simulink model "Vorlage_Prozessgut_Gruppen3"  (R2023b)
settings: Solver=ode3  StartTime=0.0  StopTime=200  FixedStep=0.01  RelTol=1e-3  EnableMultiTasking=on
undefined symbols (not defined in the file): MaxFlaschen
libraries: simulink x10
settings Model: Creator=merz  LastModifiedBy=JCP
settings SolverCC: ZeroCrossAlgorithm=Non-adaptive  AlgebraicLoopSolver=TrustRegion  AutoInsertRateTranBlk=on
settings DataIOCC: LimitDataPoints=on  SaveFormat=Array  SignalLoggingSaveFormat=ModelDataLogs  ReturnWorkspaceOutputs=off  SignalLoggingName=sigsOut
settings OptimizationCC: ExpressionDepthLimit=2147483647  InitFltsAndDblsToZero=on  LifeSpan=inf
settings DebuggingCC: SaveWithParameterizedLinksMsg=none  UnderspecifiedInitializationDetection=Classic  MergeDetectMultiDrivingBlocksExec=none  SignalResolutionControl=TryResolveAllWithWarning  MultiTaskDSMMsg=warning  MultiTaskCondExecSysMsg=none  FcnCallInpInsideContextMsg=warning  UnconnectedInputMsg=warning  UnconnectedOutputMsg=warning  UnconnectedLineMsg=warning  StateNameClashWarn=warning  SFUnexpectedBacktrackingDiag=warning  SFNoUnconditionalDefaultTransitionDiag=warning  SFExecutionAtInitializationDiag=none  ArithmeticOperatorsInVariantConditions=warning
settings HardwareCC: ProdBitPerPointer=32  ProdBitPerSizeT=32  ProdBitPerPtrDiffT=32  ProdLargestAtomicFloat=None  ProdIntDivRoundTo=Undefined  ProdEndianess=Unspecified  ProdWordSize=32  ProdHWDeviceType=32-bit Generic  TargetUnknown=on
settings ModelReferenceCC: EnableRefExpFcnMdlSchedulingChecks=on  PropagateSignalLabelsOutOfModel=off
settings RTWCC: DLArmComputeVersion=19.05
settings CodeAppCC: StateflowObjectComments=on
settings GRTTargetCC: TargetFcnLib=ansi_tfl_tmw.mat  TargetLangStandard=C89/C90 (ANSI)  ModelReferenceCompliant=off  CombineOutputUpdateFcns=off  MatFileLogging=off  GRTInterface=on
settings ConfigComp: CovMetricSettings=dw  CovSaveCumulativeToWorkspaceVar=on  CovSaveSingleToWorkspaceVar=on

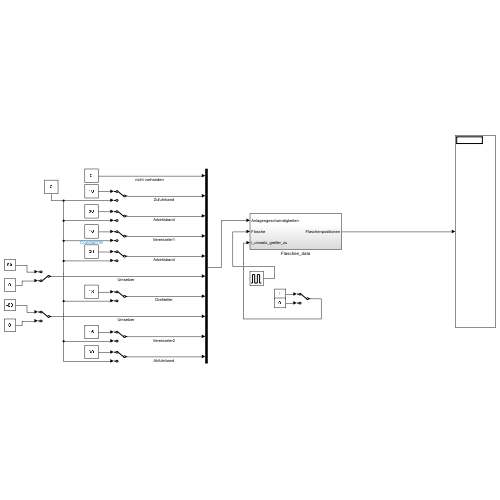
[thumbnail: Simulink's stored preview of the top-level diagram]
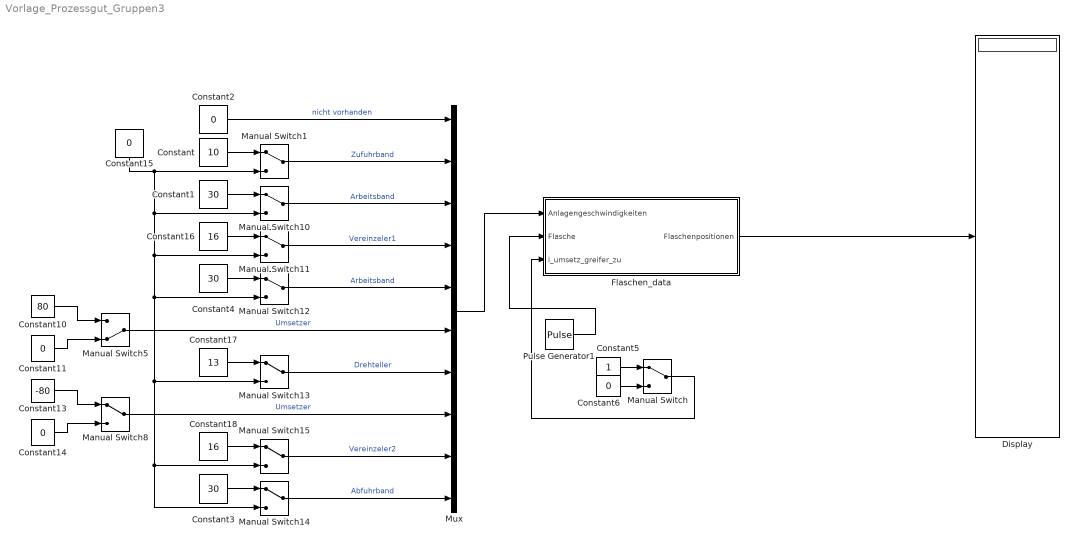
== system Vorlage_Prozessgut_Gruppen3 ==
  Constant : Constant  Value=10
  Constant1 : Constant  Value=30
  Constant10 : Constant  Value=80
  Constant{2,6,11,14..15} (5 alike) : Constant  Value=0
  Constant13 : Constant  Value=-80
  Constant16 : Constant  Value=16
  Constant17 : Constant  Value=13
  Constant18 : Constant  Value=16
  Constant3 : Constant  Value=30
  Constant4 : Constant  Value=30
  Constant5 : Constant
  Display : Display
  Flaschen_data : Subsystem
  Manual Switch{,1,8,10..15} (9 alike) : ManualSwitch
  Manual Switch5 : ManualSwitch  CurrentSetting=0
  Mux : Mux  Inputs=10
  Pulse Generator1 : DiscretePulseGenerator  PulseType=Time based  Period=15  PulseWidth=5
  wires:
  Constant17/1 -> Manual Switch13/1
  Manual Switch12/1 -> Mux/5  "Arbeitsband"
  Constant16/1 -> Manual Switch11/1
  Constant10/1 -> Manual Switch5/1
  Constant14/1 -> Manual Switch8/2
  Constant1/1 -> Manual Switch10/1
  Constant2/1 -> Mux/1  "nicht vorhanden"
  Manual Switch10/1 -> Mux/3  "Arbeitsband"
  Constant11/1 -> Manual Switch5/2
  Constant/1 -> Manual Switch1/1
  Constant13/1 -> Manual Switch8/1
  Manual Switch8/1 -> Mux/8  "Umsetzer"
  Manual Switch5/1 -> Mux/6  "Umsetzer"
  Manual Switch15/1 -> Mux/9  "Vereinzeler2"
  Constant3/1 -> Manual Switch14/1
  Constant4/1 -> Manual Switch12/1
  Manual Switch1/1 -> Mux/2  "Zufuhrband"
  Mux/1 -> Flaschen_data/1(Anlagengeschwindigkeiten)
  Manual Switch11/1 -> Mux/4  "Vereinzeler1"
  Manual Switch13/1 -> Mux/7  "Drehteller"
  Manual Switch14/1 -> Mux/10  "Abfuhrband"
  Constant18/1 -> Manual Switch15/1
  Constant15/1 -> Manual Switch12/2, Manual Switch13/2, Manual Switch15/2, Manual Switch14/2, Manual Switch11/2, Manual Switch10/2, Manual Switch1/2
  Constant6/1 -> Manual Switch/2
  Pulse Generator1/1 -> Flaschen_data/2(Flasche)
  Constant5/1 -> Manual Switch/1
  Manual Switch/1 -> Flaschen_data/3(i_umsetz_greifer_zu)
  Flaschen_data/1(Flaschenpositionen) -> Display/1

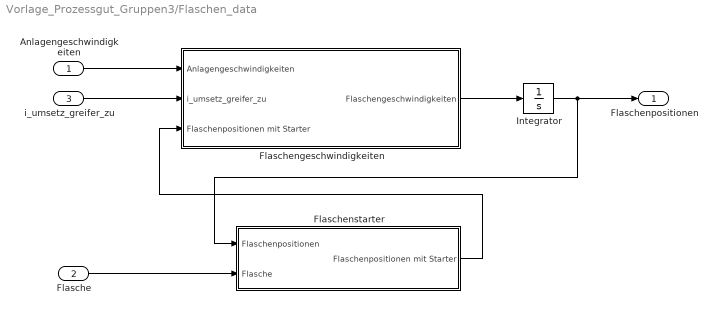
== system Vorlage_Prozessgut_Gruppen3/Flaschen_data ==
  Anlagengeschwindigkeiten : Inport
  Flasche : Inport  Port=2
  i_umsetz_greifer_zu : Inport  Port=3
  Flaschengeschwindigkeiten : Subsystem
  Flaschenstarter : Subsystem
  Integrator : Integrator
  Flaschenpositionen : Outport
  wires:
  Anlagengeschwindigkeiten/1 -> Flaschengeschwindigkeiten/1(Anlagengeschwindigkeiten)
  i_umsetz_greifer_zu/1 -> Flaschengeschwindigkeiten/2(i_umsetz_greifer_zu)
  Flaschenstarter/1(Flaschenpositionen mit Starter) -> Flaschengeschwindigkeiten/3(Flaschenpositionen mit Starter)
  Flasche/1 -> Flaschenstarter/2(Flasche)
  Flaschengeschwindigkeiten/1(Flaschengeschwindigkeiten) -> Integrator/1
  Integrator/1 -> Flaschenpositionen/1, Flaschenstarter/1(Flaschenpositionen)

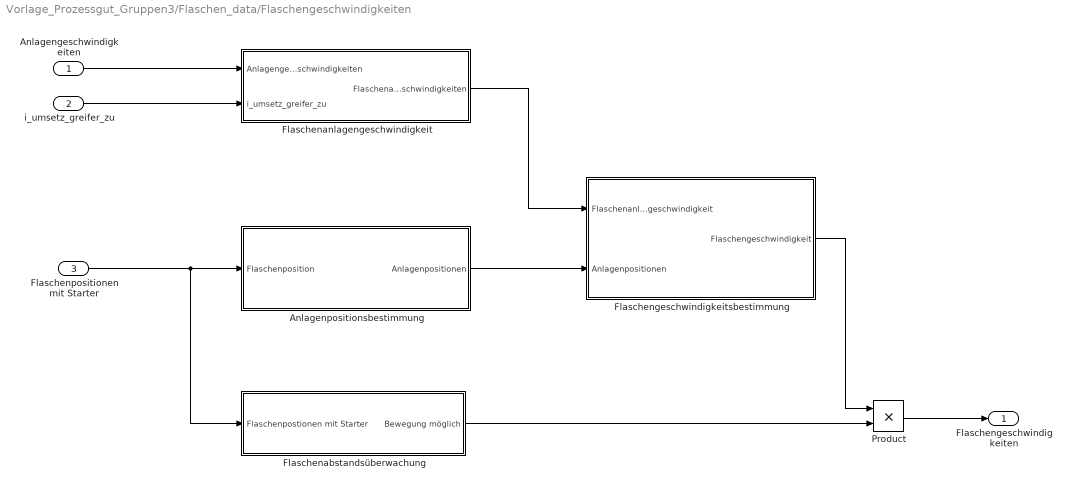
== system Vorlage_Prozessgut_Gruppen3/Flaschen_data/Flaschengeschwindigkeiten ==
  Anlagengeschwindigkeiten : Inport
  i_umsetz_greifer_zu : Inport  Port=2
  Flaschenpositionen mit Starter : Inport  Port=3
  Anlagenpositionsbestimmung : Subsystem
  Flaschenabstandsüberwachung : Subsystem
  Flaschenanlagengeschwindigkeit : Subsystem
  "Flaschengeschwindigkeitsbestimmung " : Subsystem  TreatAsAtomicUnit=on
  Product : Product
  Flaschengeschwindigkeiten : Outport
  wires:
  Anlagengeschwindigkeiten/1 -> Flaschenanlagengeschwindigkeit/1(Anlagengeschwindigkeiten)
  i_umsetz_greifer_zu/1 -> Flaschenanlagengeschwindigkeit/2(i_umsetz_greifer_zu)
  Flaschenpositionen mit Starter/1 -> Flaschenabstandsüberwachung/1(Flaschenpostionen mit Starter), Anlagenpositionsbestimmung/1(Flaschenposition)
  Anlagenpositionsbestimmung/1(Anlagenpositionen) -> "Flaschengeschwindigkeitsbestimmung "/2(Anlagenpositionen)
  Flaschenanlagengeschwindigkeit/1(Flaschenanlagengeschwindigkeiten) -> "Flaschengeschwindigkeitsbestimmung "/1(Flaschenanlagengeschwindigkeit)
  Flaschenabstandsüberwachung/1(Bewegung möglich) -> Product/2
  "Flaschengeschwindigkeitsbestimmung "/1(Flaschengeschwindigkeit) -> Product/1
  Product/1 -> Flaschengeschwindigkeiten/1

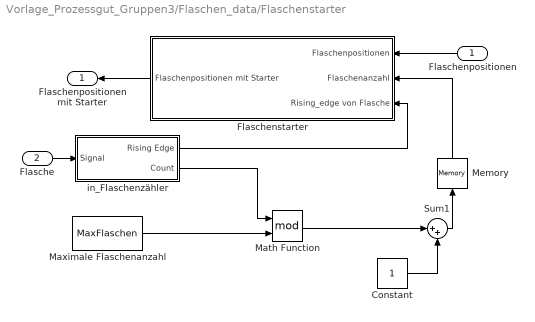
== system Vorlage_Prozessgut_Gruppen3/Flaschen_data/Flaschenstarter ==
  Flaschenpositionen : Inport
  Flasche : Inport  Port=2
  Constant : Constant  OutDataTypeStr=uint16
  Flaschenstarter : Subsystem
  Math Function : Math  Operator=mod  SignedPower=on
  Maximale Flaschenanzahl : Constant  Value=MaxFlaschen  OutDataTypeStr=uint16
  Memory : Memory  InitialCondition=1
  Sum1 : Sum  Inputs=|++  SaturateOnIntegerOverflow=on
  in_Flaschenzähler : Subsystem
  Flaschenpositionen mit Starter : Outport
  wires:
  in_Flaschenzähler/2(Count) -> Math Function/1
  Maximale Flaschenanzahl/1 -> Math Function/2
  Math Function/1 -> Sum1/1
  in_Flaschenzähler/1(Rising Edge) -> Flaschenstarter/3(Rising_edge von Flasche)
  Sum1/1 -> Memory/1
  Constant/1 -> Sum1/2
  Memory/1 -> Flaschenstarter/2(Flaschenanzahl)
  Flaschenpositionen/1 -> Flaschenstarter/1(Flaschenpositionen)
  Flaschenstarter/1(Flaschenpositionen mit Starter) -> Flaschenpositionen mit Starter/1
  Flasche/1 -> in_Flaschenzähler/1(Signal)

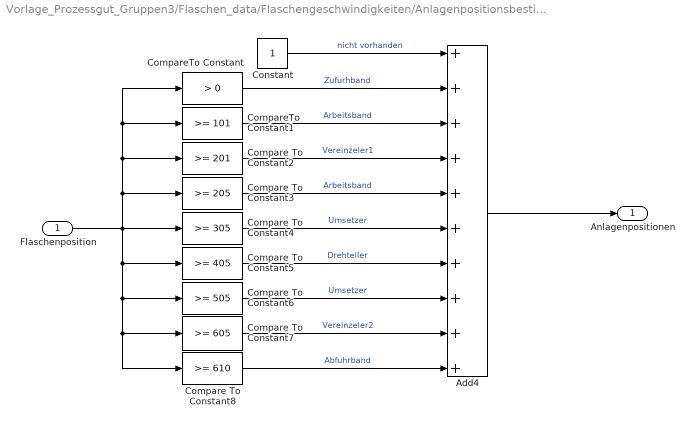
== system Vorlage_Prozessgut_Gruppen3/Flaschen_data/Flaschengeschwindigkeiten/Anlagenpositionsbestimmung ==
  Flaschenposition : Inport
  Add4 : Sum  Inputs=++++++++++
  Compare To Constant2 : simulink/Logic and Bit Operations/Compare To Constant  relop=>=  const=201  OutDataTypeStr=uint8  ZeroCross=off
  Compare To Constant3 : simulink/Logic and Bit Operations/Compare To Constant  relop=>=  const=205  OutDataTypeStr=uint8  ZeroCross=off
  Compare To Constant4 : simulink/Logic and Bit Operations/Compare To Constant  relop=>=  const=305  OutDataTypeStr=uint8  ZeroCross=off
  Compare To Constant5 : simulink/Logic and Bit Operations/Compare To Constant  relop=>=  const=405  OutDataTypeStr=uint8  ZeroCross=off
  Compare To Constant6 : simulink/Logic and Bit Operations/Compare To Constant  relop=>=  const=505  OutDataTypeStr=uint8  ZeroCross=off
  Compare To Constant7 : simulink/Logic and Bit Operations/Compare To Constant  relop=>=  const=605  OutDataTypeStr=uint8  ZeroCross=off
  Compare To Constant8 : simulink/Logic and Bit Operations/Compare To Constant  relop=>=  const=610  OutDataTypeStr=uint8  ZeroCross=off
  CompareTo Constant : simulink/Logic and Bit Operations/Compare To Constant  relop=>  const=0  OutDataTypeStr=uint8  ZeroCross=off
  CompareTo Constant1 : simulink/Logic and Bit Operations/Compare To Constant  relop=>=  const=101  OutDataTypeStr=uint8  ZeroCross=off
  Constant : Constant
  Anlagenpositionen : Outport
  wires:
  Add4/1 -> Anlagenpositionen/1
  Flaschenposition/1 -> Compare To Constant3/1, Compare To Constant2/1, CompareTo Constant1/1, CompareTo Constant/1, Compare To Constant8/1, Compare To Constant7/1, Compare To Constant6/1, Compare To Constant5/1, Compare To Constant4/1
  Constant/1 -> Add4/1  "nicht vorhanden"
  CompareTo Constant/1 -> Add4/2  "Zufurhband"
  CompareTo Constant1/1 -> Add4/3  "Arbeitsband"
  Compare To Constant2/1 -> Add4/4  "Vereinzeler1"
  Compare To Constant3/1 -> Add4/5  "Arbeitsband"
  Compare To Constant4/1 -> Add4/6  "Umsetzer"
  Compare To Constant5/1 -> Add4/7  "Drehteller"
  Compare To Constant6/1 -> Add4/8  "Umsetzer"
  Compare To Constant7/1 -> Add4/9  "Vereinzeler2"
  Compare To Constant8/1 -> Add4/10  "Abfuhrband"

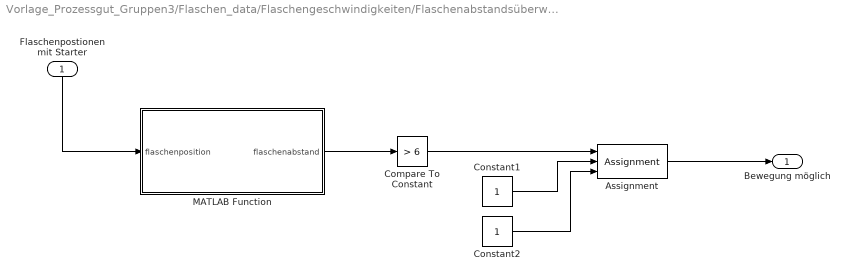
== system Vorlage_Prozessgut_Gruppen3/Flaschen_data/Flaschengeschwindigkeiten/Flaschenabstandsüberwachung ==
  Flaschenpostionen mit Starter : Inport
  Assignment : Assignment  IndexOptions=Index vector (port)  Indices=1  OutputSizes=[1]
  Compare To Constant : simulink/Logic and Bit Operations/Compare To Constant  relop=>  const=6  OutDataTypeStr=boolean  ZeroCross=off
  Constant1 : Constant  OutDataTypeStr=boolean
  Constant2 : Constant  OutDataTypeStr=int8
  MATLAB Function : MATLAB Function  TreatAsAtomicUnit=on
  Bewegung möglich : Outport
  wires:
  Constant1/1 -> Assignment/2
  Flaschenpostionen mit Starter/1 -> MATLAB Function/1(flaschenposition)
  Constant2/1 -> Assignment/3
  Compare To Constant/1 -> Assignment/1
  Assignment/1 -> Bewegung möglich/1
  MATLAB Function/1(flaschenabstand) -> Compare To Constant/1

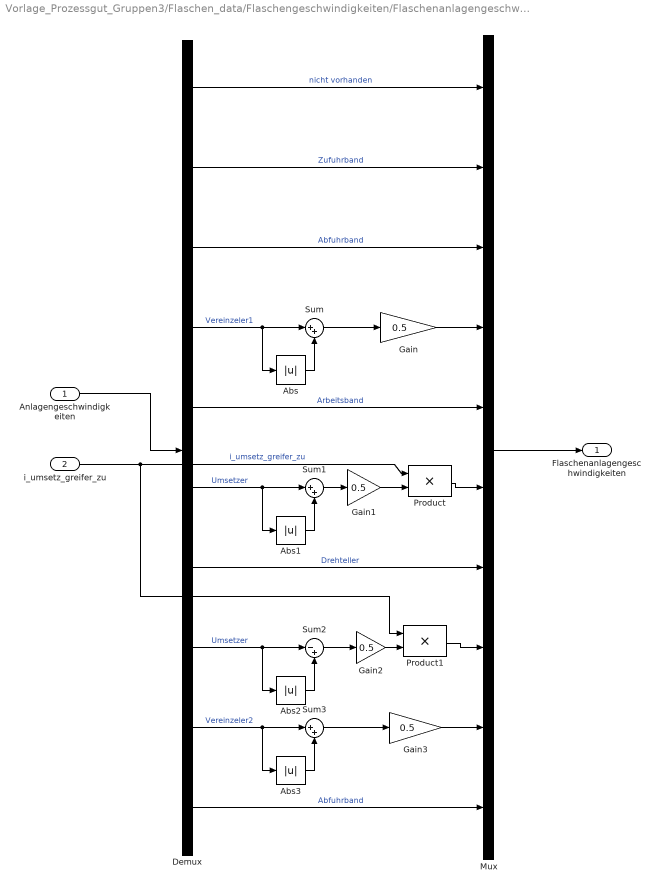
== system Vorlage_Prozessgut_Gruppen3/Flaschen_data/Flaschengeschwindigkeiten/Flaschenanlagengeschwindigkeit ==
  Anlagengeschwindigkeiten : Inport
  i_umsetz_greifer_zu : Inport  Port=2
  Abs{,1..3} (4 alike) : Abs
  Demux : Demux  Outputs=10
      settings: DisplayOption=none
  Gain{,1..3} (4 alike) : Gain  Gain=0.5  SaturateOnIntegerOverflow=on  OutDataTypeStr=Inherit: Same as input  ParamDataTypeStr=Inherit: Same as input
  Mux : Mux  Inputs=10
  Product : Product  OutDataTypeStr=double  SaturateOnIntegerOverflow=on
  Product1 : Product  OutDataTypeStr=double  SaturateOnIntegerOverflow=on
  Sum : Sum  Inputs=|++  SaturateOnIntegerOverflow=on
  Sum1 : Sum  Inputs=|++  SaturateOnIntegerOverflow=on
  Sum2 : Sum  Inputs=|-+  SaturateOnIntegerOverflow=on
  Sum3 : Sum  Inputs=|++  SaturateOnIntegerOverflow=on
  Flaschenanlagengeschwindigkeiten : Outport
  wires:
  Gain3/1 -> Mux/9
  i_umsetz_greifer_zu/1 -> Product1/1, Product/1  "i_umsetz_greifer_zu"
  Abs/1 -> Sum/2
  Sum1/1 -> Gain1/1
  Demux/1 -> Mux/1  "nicht vorhanden"
  Demux/10 -> Mux/10  "Abfuhrband"
  Abs3/1 -> Sum3/2
  Abs1/1 -> Sum1/2
  Sum/1 -> Gain/1
  Demux/7 -> Mux/7  "Drehteller"
  Gain/1 -> Mux/4
  Demux/3 -> Mux/3  "Abfuhrband"
  Demux/8 -> Sum2/1, Abs2/1  "Umsetzer"
  Mux/1 -> Flaschenanlagengeschwindigkeiten/1
  Abs2/1 -> Sum2/2
  Demux/9 -> Sum3/1, Abs3/1  "Vereinzeler2"
  Gain1/1 -> Product/2
  Demux/2 -> Mux/2  "Zufuhrband"
  Demux/4 -> Sum/1, Abs/1  "Vereinzeler1"
  Gain2/1 -> Product1/2
  Sum2/1 -> Gain2/1
  Product1/1 -> Mux/8
  Anlagengeschwindigkeiten/1 -> Demux/1
  Demux/6 -> Sum1/1, Abs1/1  "Umsetzer"
  Product/1 -> Mux/6
  Sum3/1 -> Gain3/1
  Demux/5 -> Mux/5  "Arbeitsband"

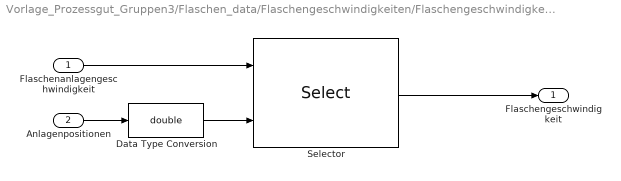
== system Vorlage_Prozessgut_Gruppen3/Flaschen_data/Flaschengeschwindigkeiten/Flaschengeschwindigkeitsbestimmung  ==
  Flaschenanlagengeschwindigkeit : Inport
  Anlagenpositionen : Inport  Port=2
  Data Type Conversion : DataTypeConversion  OutDataTypeStr=double  SaturateOnIntegerOverflow=off  RndMeth=Floor
  Selector : Selector  InputPortWidth=10  IndexOptions=Index vector (port)  Indices=[1 3]  OutputSizes=1
  Flaschengeschwindigkeit : Outport
  wires:
  Flaschenanlagengeschwindigkeit/1 -> Selector/1
  Selector/1 -> Flaschengeschwindigkeit/1
  Anlagenpositionen/1 -> Data Type Conversion/1
  Data Type Conversion/1 -> Selector/2

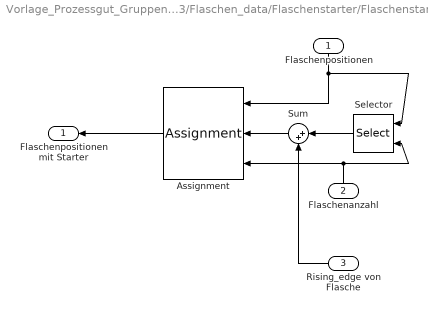
== system Vorlage_Prozessgut_Gruppen3/Flaschen_data/Flaschenstarter/Flaschenstarter ==
  Flaschenpositionen : Inport
  Flaschenanzahl : Inport  Port=2
  Rising_edge von Flasche : Inport  Port=3
  Assignment : Assignment  IndexOptions=Index vector (port)  Indices=1  OutputSizes=[1]
  Selector : Selector  InputPortWidth=MaxFlaschen  IndexOptions=Index vector (port)  Indices=[1 3]  OutputSizes=1
  Sum : Sum  Inputs=|++  OutDataTypeStr=double  RndMeth=Zero
  Flaschenpositionen mit Starter : Outport
  wires:
  Selector/1 -> Sum/1
  Sum/1 -> Assignment/2
  Flaschenanzahl/1 -> Selector/2, Assignment/3
  Flaschenpositionen/1 -> Assignment/1, Selector/1
  Assignment/1 -> Flaschenpositionen mit Starter/1
  Rising_edge von Flasche/1 -> Sum/2

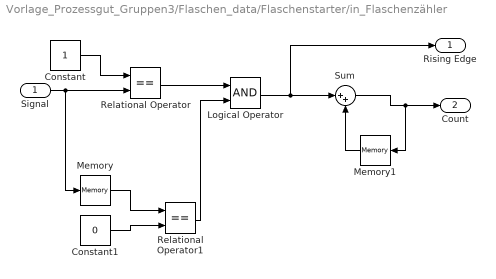
== system Vorlage_Prozessgut_Gruppen3/Flaschen_data/Flaschenstarter/in_Flaschenzähler ==
  Signal : Inport
  Constant : Constant
  Constant1 : Constant  Value=0
  Logical Operator : Logic  AllPortsSameDT=off
  Memory : Memory
  Memory1 : Memory
  Relational Operator : RelationalOperator  Operator===  InputSameDT=off
  Relational Operator1 : RelationalOperator  Operator===  InputSameDT=off
  Sum : Sum  Inputs=|++  OutDataTypeStr=uint16  SaturateOnIntegerOverflow=on
  Rising Edge : Outport
  Count : Outport  Port=2
  wires:
  Signal/1 -> Relational Operator/2, Memory/1
  Constant/1 -> Relational Operator/1
  Relational Operator/1 -> Logical Operator/1
  Constant1/1 -> Relational Operator1/2
  Memory/1 -> Relational Operator1/1
  Relational Operator1/1 -> Logical Operator/2
  Logical Operator/1 -> Sum/1, Rising Edge/1
  Memory1/1 -> Sum/2
  Sum/1 -> Count/1, Memory1/1

== matlab function Vorlage_Prozessgut_Gruppen3/Flaschen_data/Flaschengeschwindigkeiten/Flaschenabstandsüberwachung/MATLAB Function ==
  data: flaschenposition input; flaschenabstand output
function flaschenabstand = fcn(flaschenposition)

flaschenabstand = circshift(flaschenposition,1) - flaschenposition;

end
